simulink library "INT_Brk_DD"  (R2016b)
settings: Solver=VariableStepAuto  StartTime=0.0  StopTime=10.0  RelTol=1e-3
settings Model: Creator=bianxuyin  LastModifiedBy=bianxuyin

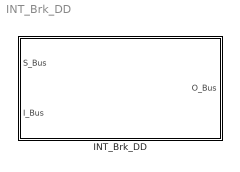
== system INT_Brk_DD ==
  INT_Brk_DD : Subsystem

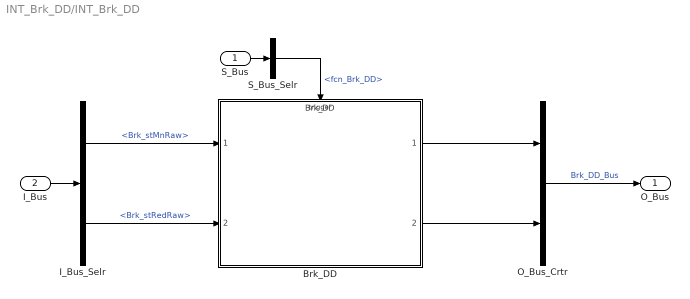
== system INT_Brk_DD/INT_Brk_DD ==
  S_Bus : Inport
  I_Bus : Inport  Port=2
  Brk_DD : ModelReference  ModelNameDialog=Brk_DD  SimulationMode=Normal  ModelReferenceVersion=1.8  TriggerPortName=function  TriggerPortTriggerType=function-call  TriggerPortStatesWhenEnabling=held
  I_Bus_Selr : BusSelector  OutputSignals=Brk_stMnRaw,Brk_stRedRaw
  O_Bus_Crtr : BusCreator  Inputs=2
  S_Bus_Selr : BusSelector  OutputSignals=fcn_Brk_DD
  O_Bus : Outport
  wires:
  S_Bus_Selr/1 -> Brk_DD/Trigger  "<fcn_Brk_DD>"
  S_Bus/1 -> S_Bus_Selr/1
  I_Bus/1 -> I_Bus_Selr/1
  I_Bus_Selr/1 -> Brk_DD/1  "<Brk_stMnRaw>"
  I_Bus_Selr/2 -> Brk_DD/2  "<Brk_stRedRaw>"
  O_Bus_Crtr/1 -> O_Bus/1  "Brk_DD_Bus"
  Brk_DD/1 -> O_Bus_Crtr/1
  Brk_DD/2 -> O_Bus_Crtr/2
